simulink model "hinfNL"  (R2022b)
settings: Solver=VariableStepAuto  StartTime=0.0  StopTime=50  RelTol=1e-3
values from neighbouring files (symbols this model uses):
  d1 = 0.13075    [TF.mat]
  d2 = 0.05075    [TF.mat]
  DZ = 3    [TF.mat]
  I = 0.00015    [TF.mat]
  km = 0.001118    [TF.mat]
  MAX_PWM = 80    [TF.mat]
  miu = 0.0005001    [TF.mat]
  wb = 0.105948    [TF.mat]
  wcp = 0.014145    [TF.mat]
  wm = 0.030411    [TF.mat]
undefined symbols (not defined in the file or in its folder): DirectCMD, HinfDiscrete, t1, t2
libraries: simulink x1
settings Model: Creator=andre  LastModifiedBy=felip
settings SolverCC: AlgebraicLoopSolver=TrustRegion
settings DebuggingCC: UnconnectedInputMsg=warning  UnconnectedOutputMsg=warning  UnconnectedLineMsg=warning  SFMachineParentedDataDiag=warning
settings ModelReferenceCC: EnableRefExpFcnMdlSchedulingChecks=on
settings RTWCC: DLArmComputeVersion=19.05

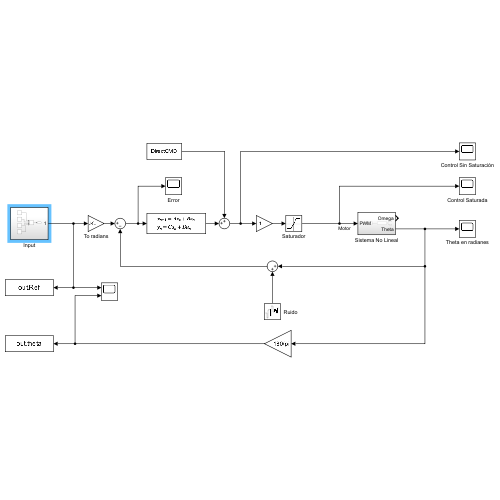
[thumbnail: Simulink's stored preview of the top-level diagram]
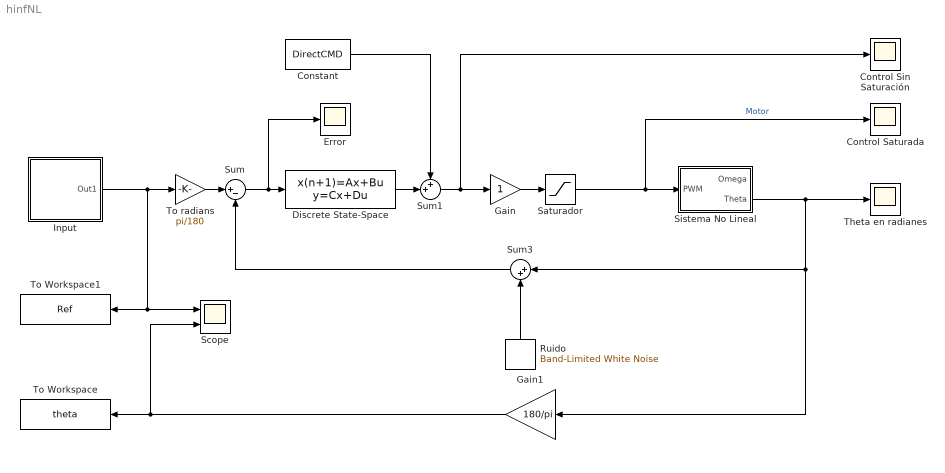
== system hinfNL ==
  Constant : Constant  Value=DirectCMD
  Control Saturada : Scope
  Control Sin Saturación : Scope
  Discrete State-Space : DiscreteStateSpace  A=HinfDiscrete.A  B=HinfDiscrete.B  C=HinfDiscrete.C  D=HinfDiscrete.D  SampleTime=2.5e-3
  Error : Scope
  Gain : Gain
  Gain1 : Gain  Gain=180/pi
  Input : Subsystem
  Ruido : simulink/Sources/Band-Limited White Noise  Cov=[0.0001]  Ts=2.5e-3  seed=[23341]
  Saturador : Saturate  UpperLimit=100  LowerLimit=0
  Scope : Scope  NumInputPorts=2
  Sistema No Lineal : Subsystem
  Sum : Sum  Inputs=|+-
  Sum1 : Sum  Inputs=++|
  Sum3 : Sum  Inputs=|++
  Theta en radianes : Scope
  To Workspace : ToWorkspace  VariableName=theta  SaveFormat=Timeseries  SampleTime=-1
  To Workspace1 : ToWorkspace  VariableName=Ref  SaveFormat=Timeseries  SampleTime=-1
  To radians : Gain  Gain=pi/180
  wires:
  Sum/1 -> Error/1, Discrete State-Space/1
  Sum3/1 -> Sum/2
  Ruido/1 -> Sum3/2
  Saturador/1 -> Control Saturada/1, Sistema No Lineal/1(PWM)  "Motor"
  To radians/1 -> Sum/1
  Gain1/1 -> To Workspace/1, Scope/2
  Sistema No Lineal/2(Theta) -> Gain1/1, Sum3/1, Theta en radianes/1
  Sum1/1 -> Control Sin Saturación/1, Gain/1
  Constant/1 -> Sum1/1
  Input/1(Out1) -> To radians/1, To Workspace1/1, Scope/1
  Discrete State-Space/1 -> Sum1/2
  Gain/1 -> Saturador/1

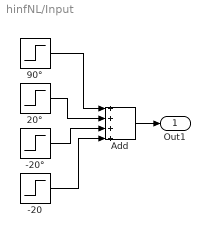
== system hinfNL/Input ==
  -20 : Step  Time=t2  After=5  SampleTime=0
  -20° : Step  Time=t1  After=-15  SampleTime=0
  20° : Step  Time=20  After=4  SampleTime=0
  90° : Step  Time=0  After=85  SampleTime=0
  Add : Sum  Inputs=++++
  Out1 : Outport
  wires:
  Add/1 -> Out1/1
  20°/1 -> Add/2
  -20/1 -> Add/4
  90°/1 -> Add/1
  -20°/1 -> Add/3

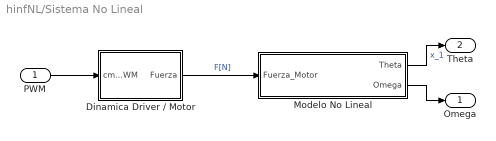
== system hinfNL/Sistema No Lineal ==
  PWM : Inport
  Dinamica Driver / Motor : Subsystem
  Modelo No Lineal : Subsystem
  Omega : Outport
  Theta : Outport  Port=2
  wires:
  PWM/1 -> Dinamica Driver / Motor/1(cmd_PWM)
  Dinamica Driver / Motor/1(Fuerza) -> Modelo No Lineal/1(Fuerza_Motor)  "F[N]"
  Modelo No Lineal/1(Theta) -> Theta/1  "x_1"
  Modelo No Lineal/2(Omega) -> Omega/1

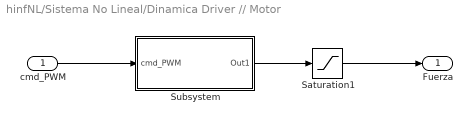
== system hinfNL/Sistema No Lineal/Dinamica Driver // Motor ==
  cmd_PWM : Inport
  Saturation1 : Saturate  UpperLimit=MAX_PWM  ZeroCross=off
  Subsystem : Subsystem
  Fuerza : Outport
  wires:
  Saturation1/1 -> Fuerza/1
  cmd_PWM/1 -> Subsystem/1(cmd_PWM)
  Subsystem/1(Out1) -> Saturation1/1

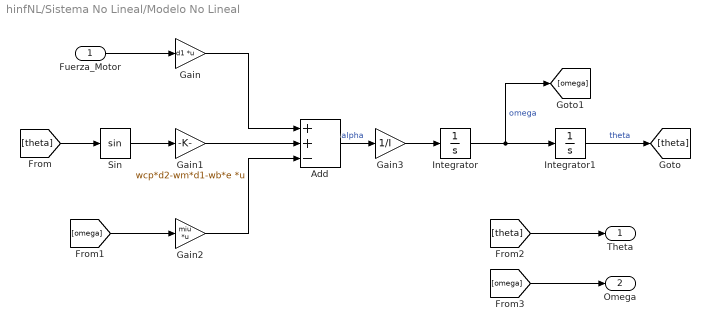
== system hinfNL/Sistema No Lineal/Modelo No Lineal ==
  Fuerza_Motor : Inport
  Add : Sum  Inputs=++-
  Gain : Gain  Gain=d1  Multiplication=Matrix(K*u)
  Gain1 : Gain  Gain=wcp*d2-wm*d1-wb*e  Multiplication=Matrix(K*u)
  Gain2 : Gain  Gain=miu  Multiplication=Matrix(K*u)
  Gain3 : Gain  Gain=1/I
  Integrator : Integrator  ZeroCross=off
  Integrator1 : Integrator  InitialCondition=85*pi/180  ZeroCross=off
  Sin : Trigonometry
  Theta : Outport
  Omega : Outport  Port=2
  wires:
  [omega] -> Omega/1
  Gain1/1 -> Add/2
  Integrator/1 -> [omega], Integrator1/1  "omega"
  Fuerza_Motor/1 -> Gain/1
  Integrator1/1 -> [theta]  "theta"
  Gain2/1 -> Add/3
  Gain/1 -> Add/1
  Add/1 -> Gain3/1  "alpha"
  [theta] -> Sin/1
  [omega] -> Gain2/1
  [theta] -> Theta/1
  Sin/1 -> Gain1/1
  Gain3/1 -> Integrator/1

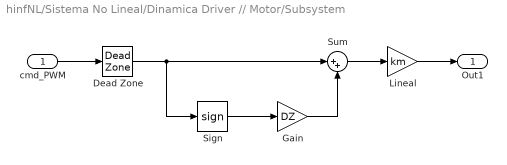
== system hinfNL/Sistema No Lineal/Dinamica Driver // Motor/Subsystem ==
  cmd_PWM : Inport
  Dead Zone : DeadZone  LowerValue=-DZ  UpperValue=DZ  ZeroCross=off
  Gain : Gain  Gain=DZ
  Lineal : Gain  Gain=km
  Sign : Signum  ZeroCross=off
  Sum : Sum  Inputs=|++
  Out1 : Outport
  wires:
  cmd_PWM/1 -> Dead Zone/1
  Dead Zone/1 -> Sum/1, Sign/1
  Sum/1 -> Lineal/1
  Sign/1 -> Gain/1
  Gain/1 -> Sum/2
  Lineal/1 -> Out1/1
